simulink model "modelofinal"  (R2022b)
settings: Solver=VariableStepAuto  StartTime=0.0  StopTime=100  RelTol=1e-3
settings Model: Creator=levis  LastModifiedBy=levis

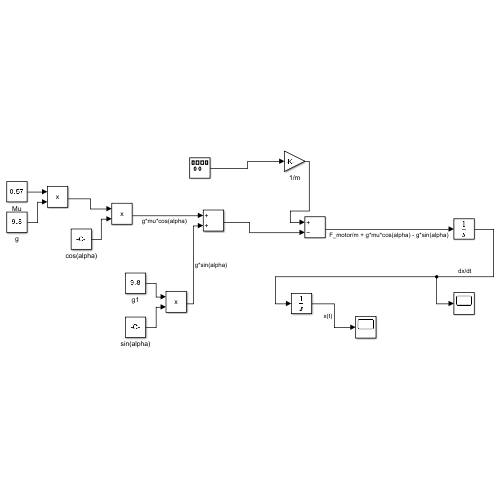
[thumbnail: Simulink's stored preview of the top-level diagram]
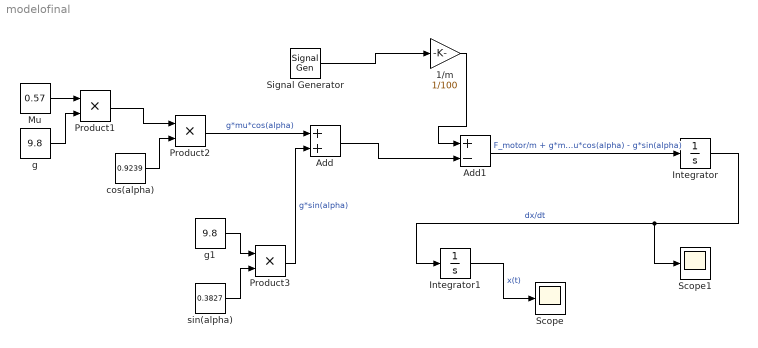
== system modelofinal ==
  1/m : Gain  Gain=1/100
  Add : Sum
  Add1 : Sum  Inputs=+-
  Integrator : Integrator
  Integrator1 : Integrator
  Mu : Constant  Value=0.57
  Product1 : Product
  Product2 : Product
  Product3 : Product
  Scope : Scope
  Scope1 : Scope
  Signal Generator : SignalGenerator  Units=rad/sec
  cos(alpha) : Constant  Value=0.9239
  g : Constant  Value=9.8
  g1 : Constant  Value=9.8
  sin(alpha) : Constant  Value=0.3827
  wires:
  Mu/1 -> Product1/1
  g/1 -> Product1/2
  Product1/1 -> Product2/1
  cos(alpha)/1 -> Product2/2
  Product2/1 -> Add/1  "g*mu*cos(alpha)"
  g1/1 -> Product3/1
  sin(alpha)/1 -> Product3/2
  Product3/1 -> Add/2  "g*sin(alpha)"
  Add/1 -> Add1/2
  Add1/1 -> Integrator/1  "F_motor/m + g*mu*cos(alpha) - g*sin(alpha)"
  Integrator/1 -> Scope1/1, Integrator1/1  "dx/dt"
  Integrator1/1 -> Scope/1  "x(t)"
  Signal Generator/1 -> 1/m/1
  1/m/1 -> Add1/1
